simulink model "mpc_sim"  (R2023a)
settings: Solver=VariableStepAuto  StartTime=0.0  StopTime=3  RelTol=1e-3
values from neighbouring files (symbols this model uses):
  B_tilda = [sysdis.B(1) Bw_bar(1,1) Bw_bar(1,2); sysdis.B(2) Bw_bar(2,1) Bw_bar(2,2)]    [motor.m]
  D_tilda = [0 0 0 ; 0 0 0]    [motor.m]
  N = 10    [motor.m]    (also in motor_mpc.m; mpc_unconstrained.m)
  Q_LQ = eye(2)    [motor.m]
  R_LQ = 1    [motor.m]
  sysdis = c2d(sys,Ts)    [motor.m]
  Ts = 0.001    [parameters.m]
  u_max = 12    [constraints.m]
  u_min = 0    [constraints.m]
  uBar = -(A(1,1)*(-A(2,2)*nref/A(2,1)) + A(1,2)*nref)*L    [motor.m]
  w = [1 1]'    [parameters.m]
  x0 = [0.2 70.3]'    [motor.m]
  yref = [iref nref]'    [motor.m]
undefined symbols (not defined in the file or in its folder): motor_mpc, Sd
settings Model: Creator=teora  LastModifiedBy=teora

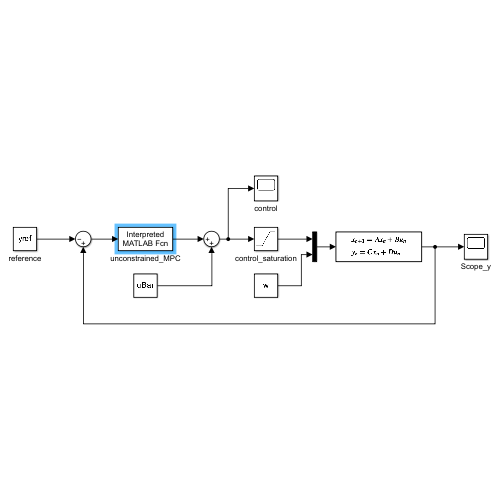
[thumbnail: Simulink's stored preview of the top-level diagram]
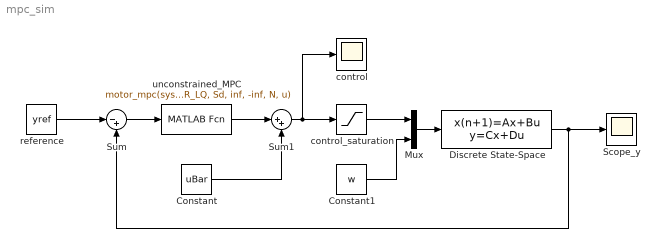
== system mpc_sim ==
  Constant : Constant  Value=uBar
  Constant1 : Constant  Value=w
  Discrete State-Space : DiscreteStateSpace  A=sysdis.A  B=B_tilda  C=sysdis.C  D=D_tilda  InitialCondition=x0  SampleTime=Ts
  Mux : Mux  Inputs=2
  Scope_y : Scope
  Sum : Sum  Inputs=|-+
  Sum1 : Sum  Inputs=|++
  control : Scope
  control_saturation : Saturate  UpperLimit=u_max  LowerLimit=u_min
  reference : Constant  Value=yref
  unconstrained_MPC : MATLABFcn  MATLABFcn=motor_mpc(sysdis.A, sysdis.B, Q_LQ, R_LQ, Sd, inf, -inf, N, u)  OutputDimensions=1
  wires:
  reference/1 -> Sum/1
  Discrete State-Space/1 -> Scope_y/1, Sum/2
  Sum/1 -> unconstrained_MPC/1
  Sum1/1 -> control/1, control_saturation/1
  Constant/1 -> Sum1/2
  unconstrained_MPC/1 -> Sum1/1
  Mux/1 -> Discrete State-Space/1
  control_saturation/1 -> Mux/1
  Constant1/1 -> Mux/2
